simulink model "model_6DOF"  (R2021a)
settings: Solver=VariableStepAuto  StartTime=0.0  StopTime=1000
values from neighbouring files (symbols this model uses):
  ae = 400    [main.m]
  C20 = -0.1    [main.m]
  C22 = 0.04    [main.m]
  eps_d = zeros(6,1)    [main.m]
  eps_d_dot = zeros(6,1)    [main.m]
  eps_r0 = [-0.06 0.05 0.09 -1 2 1.5]'    [main.m]
  eps_rb0 = [ang_vel_0_rb;v_rb]    [main.m]
  g_d = g_rh    [main.m]
  g_r0 = [A_r0 r_r0; zeros(1,3) 1]    [main.m]
  g_rb0 = [A_rb0 r_rb; zeros(1,3) 1]    [main.m]
  I_bold_sc = [I_sc zeros(3,3); zeros(3,3) m_sc*eye(3)]    [main.m]
  I_sc = [2 0 0; 0 1 0; 0 0 1.6].*10^3    [main.m]
  Kd = 0.04*eye(6)    [main.m]
  Kp = 4*(10^(-4))*eye(6)    [main.m]
  m_sc = 1e03    (= 1000)    [main.m]
  mu = 94    [main.m]
settings Model: Creator=danie  LastModifiedBy=danie

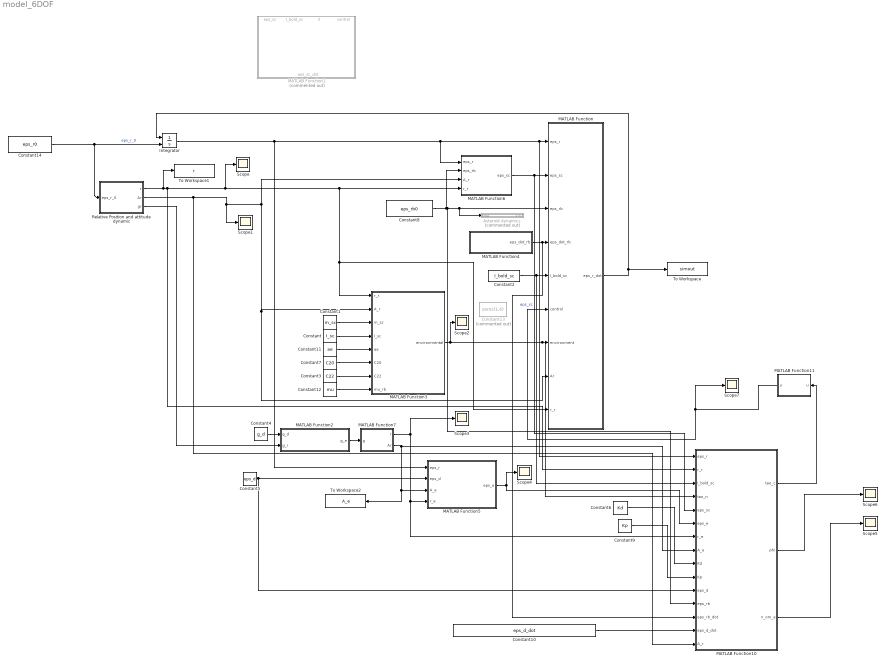
== system model_6DOF ==
  Asteroid dynamics : Subsystem  Commented=on
  Constant : Constant  Value=I_sc
  Constant1 : Constant  Value=m_sc
  Constant10 : Constant  Value=eps_d_dot
  Constant11 : Constant  Value=ae
  Constant12 : Constant  Value=mu
  Constant13 : Constant  Commented=on  Value=zeros(1,6)
  Constant14 : Constant  Value=eps_r0
  Constant2 : Constant  Value=I_bold_sc
  Constant3 : Constant  Value=C22
  Constant4 : Constant  Value=g_d
  Constant5 : Constant  Value=eps_d
  Constant6 : Constant  Value=Kd
  Constant7 : Constant  Value=C20
  Constant8 : Constant  Value=eps_rb0
  Constant9 : Constant  Value=Kp
  Integrator : Integrator  InitialConditionSource=external
  MATLAB Function : MATLAB Function  TreatAsAtomicUnit=on
  MATLAB Function1 : MATLAB Function  Commented=on  TreatAsAtomicUnit=on
  MATLAB Function10 : MATLAB Function  TreatAsAtomicUnit=on
  MATLAB Function11 : MATLAB Function  TreatAsAtomicUnit=on
  MATLAB Function2 : MATLAB Function  TreatAsAtomicUnit=on
  MATLAB Function3 : MATLAB Function  TreatAsAtomicUnit=on
  MATLAB Function4 : MATLAB Function  TreatAsAtomicUnit=on
  MATLAB Function5 : MATLAB Function  TreatAsAtomicUnit=on
  MATLAB Function6 : MATLAB Function  TreatAsAtomicUnit=on
  MATLAB Function7 : MATLAB Function  TreatAsAtomicUnit=on
  Relative Position and attitude dynamic : Subsystem
  Scope{,1..7} (8 alike) : Scope
  To Workspace : ToWorkspace  VariableName=simout  SaveFormat=Timeseries  SampleTime=-1
  To Workspace1 : ToWorkspace  VariableName=r  SaveFormat=Timeseries  SampleTime=-1
  To Workspace2 : ToWorkspace  VariableName=A_e  SaveFormat=Timeseries  SampleTime=-1
  wires:
  MATLAB Function/1(eps_r_dot) -> Integrator/1, To Workspace/1
  Constant14/1 -> Integrator/2, Relative Position and attitude dynamic/1(eps_r_0)  "eps_r_0"
  MATLAB Function3/1(environmental) -> MATLAB Function10/4(tao_n), MATLAB Function/7(environment), Scope2/1
  Constant2/1 -> MATLAB Function/5(I_bold_sc), MATLAB Function10/3(I_bold_sc)
  MATLAB Function6/1(eps_sc) -> MATLAB Function/2(eps_sc), MATLAB Function10/5(eps_sc)  "eps_sc"
  MATLAB Function4/1(eps_dot_rb) -> MATLAB Function/4(eps_dot_rb), MATLAB Function10/13(eps_rb_dot)
  Constant1/1 -> MATLAB Function3/3(m_sc)
  Constant/1 -> MATLAB Function3/4(I_sc)
  Constant11/1 -> MATLAB Function3/5(ae)
  Constant7/1 -> MATLAB Function3/6(C20)
  Constant12/1 -> MATLAB Function3/8(mu_rb)
  Constant3/1 -> MATLAB Function3/7(C22)
  Constant8/1 -> MATLAB Function/3(eps_rb), Asteroid dynamics/1(Input), MATLAB Function10/12(eps_rb), MATLAB Function6/2(eps_rb)
  Relative Position and attitude dynamic/1(r) -> MATLAB Function10/2(r_r), Scope/1, MATLAB Function3/1(r_r), MATLAB Function/9(r_r), MATLAB Function6/4(r_r), To Workspace1/1
  Constant4/1 -> MATLAB Function2/1(g_d)
  Relative Position and attitude dynamic/3(gr) -> MATLAB Function2/2(g_r)
  Constant5/1 -> MATLAB Function10/11(eps_d), MATLAB Function5/2(eps_d)
  MATLAB Function2/1(g_e) -> MATLAB Function7/1(g)
  MATLAB Function7/1(r) -> MATLAB Function10/7(r_e), MATLAB Function5/4(r_e), Scope3/1
  MATLAB Function7/2(Ar) -> MATLAB Function10/8(A_e), To Workspace2/1, MATLAB Function5/3(A_e)
  MATLAB Function5/1(eps_e) -> Scope4/1, MATLAB Function10/6(eps_e)
  Constant6/1 -> MATLAB Function10/9(Kd)
  Constant9/1 -> MATLAB Function10/10(Kp)
  Constant10/1 -> MATLAB Function10/14(eps_d_dot)
  Integrator/1 -> MATLAB Function/1(eps_r), MATLAB Function10/1(eps_r), MATLAB Function6/1(eps_r), MATLAB Function5/1(eps_r)
  MATLAB Function11/1(y) -> MATLAB Function/6(control), Scope7/1
  MATLAB Function10/1(tao_c) -> MATLAB Function11/1(u)
  MATLAB Function10/2(phi) -> Scope6/1
  MATLAB Function10/3(n_om_e) -> Scope5/1
  Relative Position and attitude dynamic/2(Ar) -> MATLAB Function10/15(A_r), MATLAB Function6/3(A_r), MATLAB Function/8(Ar), MATLAB Function3/2(A_r), Scope1/1

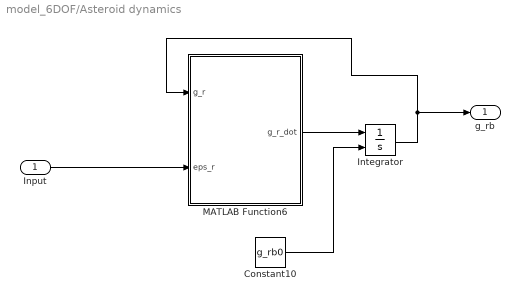
== system model_6DOF/Asteroid dynamics ==
  Input : Inport
  Constant10 : Constant  Value=g_rb0
  Integrator : Integrator  InitialConditionSource=external
  MATLAB Function6 : MATLAB Function  TreatAsAtomicUnit=on
  g_rb : Outport
  wires:
  Constant10/1 -> Integrator/2
  Input/1 -> MATLAB Function6/2(eps_r)
  MATLAB Function6/1(g_r_dot) -> Integrator/1
  Integrator/1 -> g_rb/1, MATLAB Function6/1(g_r)

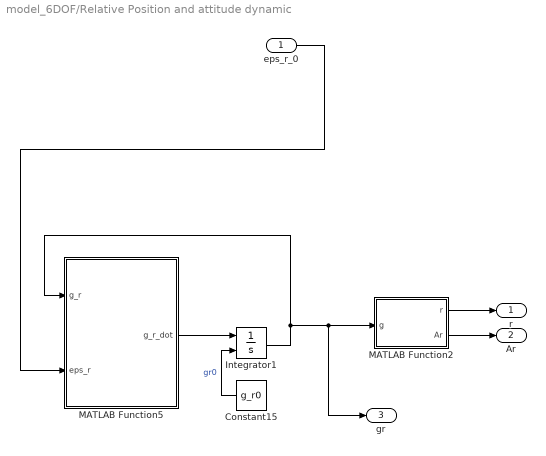
== system model_6DOF/Relative Position and attitude dynamic ==
  eps_r_0 : Inport
  Constant15 : Constant  Value=g_r0
  Integrator1 : Integrator  InitialConditionSource=external
  MATLAB Function2 : MATLAB Function  TreatAsAtomicUnit=on
  MATLAB Function5 : MATLAB Function  TreatAsAtomicUnit=on
  r : Outport
  Ar : Outport  Port=2
  gr : Outport  Port=3
  wires:
  MATLAB Function2/1(r) -> r/1
  Integrator1/1 -> gr/1, MATLAB Function2/1(g), MATLAB Function5/1(g_r)
  eps_r_0/1 -> MATLAB Function5/2(eps_r)
  Constant15/1 -> Integrator1/2  "gr0"
  MATLAB Function5/1(g_r_dot) -> Integrator1/1
  MATLAB Function2/2(Ar) -> Ar/1

== matlab function model_6DOF/MATLAB Function2 ==
  data: g_d input; g_e output; g_r input
function g_e = error_pos(g_d,g_r)
g_e=(g_d\eye(4))*g_r;

== matlab function model_6DOF/MATLAB Function5 ==
  data: eps_r input; eps_e output; eps_d input; A_e input; r_e input
function eps_e = error_eps(eps_r,eps_d,A_e,r_e)
A_inv=A_e\eye(3);
Ad_ge_inv=[A_inv zeros(3,3); lie_cross(-A_inv*r_e)*A_inv A_inv];

eps_e=eps_r-Ad_ge_inv*eps_d;

== matlab function model_6DOF/MATLAB Function7 ==
  data: g input; r output; Ar output
function [r,Ar] = g2rAr(g)
r=g(1:3,4);
Ar=g(1:3,1:3);

== matlab function model_6DOF/MATLAB Function10 ==
  data: eps_r input; r_r input; I_bold_sc input; tao_c output; tao_n input; eps_sc input; eps_e input; r_e input; A_e input; Kd input; Kp input; eps_d input; eps_rb input; eps_rb_dot input; eps_d_dot input; phi output; n_om_e output; A_r input
function [tao_c,phi,n_om_e] = control(eps_r,r_r,I_bold_sc,tao_n,eps_sc,eps_e,r_e,A_e,Kd,Kp,eps_d,eps_rb,eps_rb_dot,eps_d_dot,A_r)
ad_star_eps_sc=[-lie_cross(eps_sc(1:3)) -lie_cross(eps_sc(4:6)); zeros(3,3) -lie_cross(eps_sc(1:3))]; 


phi=acos(0.5*(trace(A_e)-1));
if phi>pi*0.9999
    phi=pi*0.9999;
end
Omega_e_cross=(phi/(2*sin(phi)))*(A_e-A_e');
A_inv_Omega_e=eye(3)-0.5*Omega_e_cross+((1/(phi^2))-(1+cos(phi)/(2*phi*sin(phi))))*Omega_e_cross*Omega_e_cross;
b_e=A_inv_Omega_e*r_e;
Omega_e=[Omega_e_cross(3,2);Omega_e_cross(1,3);Omega_e_cross(2,1)];
n_om_e=norm(Omega_e)-phi;
phi=norm(Omega_e);%%%%
ad_ne=[Omega_e_cross zeros(3,3); lie_cross(b_e) Omega_e_cross];
alfa_phi=(phi/2)*cot(phi/2);
beta_phi=((phi/2)/sin(phi/2))^2;
A_phi=(2/(phi^2))*(1-alfa_phi)+(1/(2*phi^2))*(alfa_phi-beta_phi);
B_phi=(1/(phi^4))*(1-alfa_phi)+(1/(2*phi^4))*(alfa_phi-beta_phi);
ne=[Omega_e; b_e];
G_ne=eye(6)+0.5*ad_ne+A_phi*(ad_ne^2)+B_phi*(ad_ne^4);
ne_dot=G_ne*eps_e;
Omega_e_dot=ne_dot(1:3);
b_e_dot=ne_dot(4:6);
Omega_e_dot_cross=lie_cross(Omega_e_dot);
b_e_dot_cross=lie_cross(b_e_dot);
ad_ne_dot=[Omega_e_dot_cross zeros(3,3); b_e_dot_cross Omega_e_dot_cross];
A_phi_dot=(1/(phi^3))*(1.5*alfa_phi+1.5*beta_phi+alfa_phi*beta_phi-4)*dot(Omega_e,Omega_e_dot)/phi;
B_phi_dot=(1/(phi^5))*(1.5*alfa_phi+1.5*beta_phi+alfa_phi*beta_phi-4)*dot(Omega_e,Omega_e_dot)/phi;
G_dot_ne=0.5*ad_ne_dot+A_phi_dot*(ad_ne^2)+A_phi*(ad_ne_dot*ad_ne+ad_ne*ad_ne_dot)+B_phi_dot*(ad_ne^4)+B_phi*(ad_ne_dot*(ad_ne^3)+ad_ne*ad_ne_dot*(ad_ne^2)+ad_ne^2*ad_ne_dot*ad_ne+ad_ne^3*ad_ne_dot);
ad_eps_e=[lie_cross(eps_e(1:3)) zeros(3,3); lie_cross(eps_e(4:6)) lie_cross(eps_e(1:3))];
A_e_inv=A_e\eye(3);
Ad_ge_inv=[A_e_inv zeros(3,3); lie_cross(-A_e_inv*r_e)*A_e_inv A_e_inv];
A_r_inv=A_r\eye(3);
Ad_gr_inv=[A_r_inv zeros(3,3); lie_cross(-A_r_inv*r_r)*A_r_inv A_r_inv];
ad_eps_r=[lie_cross(eps_r(1:3)) zeros(3,3); lie_cross(eps_r(4:6)) lie_cross(eps_r(1:3))];
tao_c=-ad_star_eps_sc*I_bold_sc*eps_sc-tao_n-I_bold_sc*(G_ne\eye(6))*(G_dot_ne*eps_e+Kd*ne_dot+Kp*ne)-I_bold_sc*(ad_eps_e*Ad_ge_inv*eps_d-Ad_ge_inv*eps_d_dot+ad_eps_r*Ad_gr_inv*eps_rb-Ad_gr_inv*eps_rb_dot);

== matlab function model_6DOF/MATLAB Function11 ==
  data: u input; y output
function y = limiter(u)
y=zeros(6,1);
if abs(u(4))>10
    y(4)=sign(u(4))*10;
else
    y(4)=u(4);
end
if abs(u(5))>10
    y(5)=sign(u(5))*10;
else
    y(5)=u(5);
end
if abs(u(6))>10
    y(6)=sign(u(6))*10;
else
    y(6)=u(6);
end

if abs(u(1))>10
    y(1)=sign(u(1))*10;
else
    y(1)=u(1);
end
if abs(u(2))>10
    y(2)=sign(u(2))*10;
else
    y(2)=u(2);
end
if abs(u(3))>10
    y(3)=sign(u(3))*10;
else
    y(3)=u(3);
end

== matlab function model_6DOF/MATLAB Function1 ==
  data: eps_sc input; eps_sc_dot output; I_bold_sc input; environmental input; control input
function eps_sc_dot = sc_dynamic(eps_sc,I_bold_sc,environmental,control)
ad_star_eps_sc=[-lie_cross(eps_sc(1:3)) -lie_cross(eps_sc(4:6)); zeros(3,3) -lie_cross(eps_sc(1:3))];
eps_sc_dot=ad_star_eps_sc*I_bold_sc*eps_sc+environmental+control;

== matlab function model_6DOF/MATLAB Function ==
  data: eps_r input; eps_r_dot output; eps_sc input; eps_rb input; eps_dot_rb input; I_bold_sc input; control input; environment input; Ar input; r_r input
function eps_r_dot = dynamic(eps_r,eps_sc,eps_rb,eps_dot_rb,I_bold_sc,control,environment,Ar,r_r)

ad_star_eps_sc=[-lie_cross(eps_sc(1:3)) -lie_cross(eps_sc(4:6)); zeros(3,3) -lie_cross(eps_sc(1:3))];

ad_eps_r=[lie_cross(eps_r(1:3)) zeros(3,3); lie_cross(eps_r(4:6)) lie_cross(eps_r(1:3))];

A_inv=Ar\eye(3);
Ad_gr_inv=[A_inv zeros(3,3); lie_cross(-A_inv*r_r)*A_inv A_inv];

eps_r_dot =(I_bold_sc\eye(6))*(ad_star_eps_sc*I_bold_sc*eps_sc+environment+control+I_bold_sc*(ad_eps_r*Ad_gr_inv*eps_rb-Ad_gr_inv*eps_dot_rb));

== matlab function model_6DOF/Relative Position and attitude dynamic/MATLAB Function2 ==
  data: g input; r output; Ar output
function [r,Ar] = g2rAr(g)
r=g(1:3,4);
Ar=g(1:3,1:3);

== matlab function model_6DOF/MATLAB Function3 ==
  data: r_r input; environmental output; A_r input; m_sc input; I_sc input; ae input; C20 input; C22 input; mu_rb input
function environmental = environmental(r_r, A_r,m_sc,I_sc,ae,C20,C22,mu_rb)
alfa_r=A_r(1,:)';
beta_r=A_r(2,:)';
gamma_r=A_r(3,:)';
R_r=A_r'*r_r;
R_=norm(R_r);
R_u=R_r/R_;
tao0=ae^2*C20;
tao2=ae^2*C22;
environmental_torque=(3*mu_rb/(R_^5))*cross(R_r,I_sc*R_r);
environmental_force=-(mu_rb*m_sc/(R_^2))*R_u+(3*mu_rb/(2*R_^4))*((5*R_u'*I_sc*R_u-trace(I_sc)+tao0*m_sc*(1-5*(dot(gamma_r,R_u))^2)-10*tao2*m_sc*(dot(alfa_r,R_u)^2-dot(beta_r,R_u)^2))*R_u-2*I_sc*R_u+2*tao0*m_sc*dot(gamma_r,R_u)*gamma_r+4*tao2*m_sc*(dot(alfa_r,R_u)*alfa_r-dot(beta_r,R_u)*beta_r));
environmental = [environmental_torque;environmental_force];

== matlab function model_6DOF/MATLAB Function4 ==
  data: eps_dot_rb output
function eps_dot_rb = rb_dynamic()
eps_dot_rb=zeros(1,6)';%ad_star_eps_rb*I_bold_rb*eps_rb + tao_rb;

== matlab function model_6DOF/Relative Position and attitude dynamic/MATLAB Function5 ==
  data: g_r input; g_r_dot output; eps_r input
function g_r_dot = g_dynamic(g_r,eps_r)
g_r_dot=g_r*[lie_cross(eps_r(1:3)) eps_r(4:6); zeros(1,4)];

== matlab function model_6DOF/Asteroid dynamics/MATLAB Function6 ==
  data: g_r input; g_r_dot output; eps_r input
function g_r_dot = g_dynamic(g_r,eps_r)
g_r_dot=g_r*[lie_cross(eps_r(1:3)) eps_r(4:6); zeros(1,4)];

== matlab function model_6DOF/MATLAB Function6 ==
  data: eps_r input; eps_sc output; eps_rb input; A_r input; r_r input
function eps_sc = fcn(eps_r,eps_rb, A_r,r_r)
A_inv=A_r\eye(3);
Ad_g_r_inv=[A_inv zeros(3,3); lie_cross(-A_inv*r_r)*A_inv A_inv];

eps_sc=eps_r-Ad_g_r_inv*eps_rb;
